simulink model "demo_sys"  (R2023a)
settings: Solver=VariableStepAuto  StartTime=0.0  StopTime=100  RelTol=1e-3
values from neighbouring files (symbols this model uses):
  w1_den = cell2mat(w1_den)    [demo.m]
  w1_num = cell2mat(w1_num)    [demo.m]
  w2_den = cell2mat(w2_den)    [demo.m]
  w2_num = cell2mat(w2_num)    [demo.m]
  w3_den = cell2mat(w3_den)    [demo.m]
  w3_num = cell2mat(w3_num)    [demo.m]
  w4_den = cell2mat(w4_den)    [demo.m]
  w4_num = cell2mat(w4_num)    [demo.m]
settings Model: Creator=nikit  LastModifiedBy=nikit

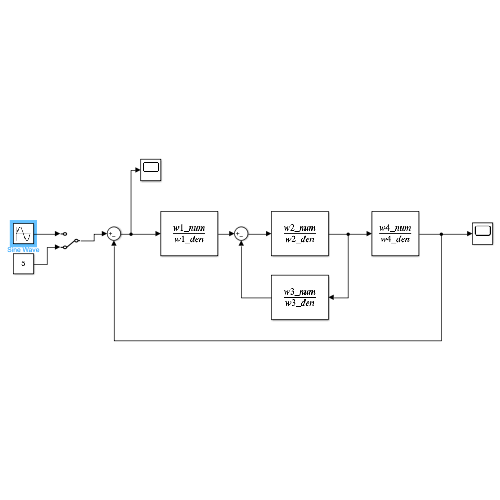
[thumbnail: Simulink's stored preview of the top-level diagram]
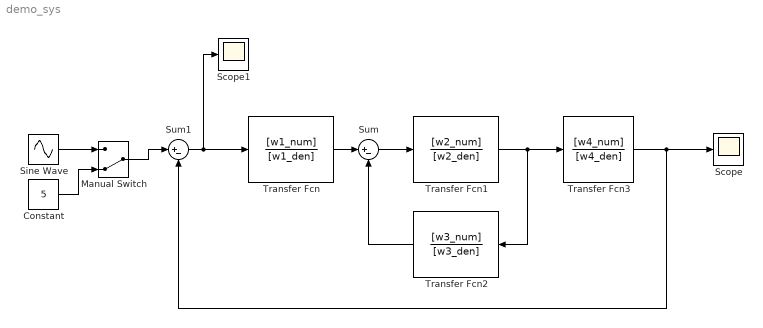
== system demo_sys ==
  Constant : Constant  Value=5
  Manual Switch : ManualSwitch  CurrentSetting=0
  Scope : Scope
  Scope1 : Scope
  Sine Wave : Sin  Amplitude=4  Frequency=0.5  SampleTime=0
  Sum : Sum  Inputs=|+-
  Sum1 : Sum  Inputs=|+-
  Transfer Fcn : TransferFcn  Numerator=[w1_num]  Denominator=[w1_den]
  Transfer Fcn1 : TransferFcn  Numerator=[w2_num]  Denominator=[w2_den]
  Transfer Fcn2 : TransferFcn  Numerator=[w3_num]  Denominator=[w3_den]
  Transfer Fcn3 : TransferFcn  Numerator=[w4_num]  Denominator=[w4_den]
  wires:
  Transfer Fcn/1 -> Sum/1
  Sum1/1 -> Scope1/1, Transfer Fcn/1
  Sum/1 -> Transfer Fcn1/1
  Transfer Fcn1/1 -> Transfer Fcn2/1, Transfer Fcn3/1
  Transfer Fcn2/1 -> Sum/2
  Transfer Fcn3/1 -> Sum1/2, Scope/1
  Sine Wave/1 -> Manual Switch/1
  Constant/1 -> Manual Switch/2
  Manual Switch/1 -> Sum1/1
